simulink model "SimLink04"  (R2021a)
settings: Solver=VariableStepAuto  StartTime=0.0  StopTime=10.0  RelTol=1e-3
libraries: dsparch4 x1, simulink_extras x1
settings Model: Creator=lefs3303  LastModifiedBy=lefs3303

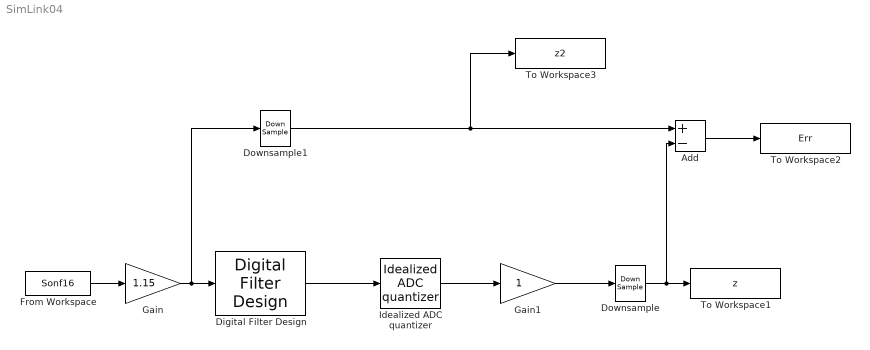
== system SimLink04 ==
  Add : Sum  Inputs=+-
  Digital Filter Design : dsparch4/Digital Filter Design  mwdsp_browser_bugfix_var=off
  Downsample : DownSample  RateOptions=Allow multirate processing
  Downsample1 : DownSample  RateOptions=Allow multirate processing
  From Workspace : FromWorkspace  VariableName=Sonf16  SampleTime=1/16000
  Gain : Gain  Gain=1.15
  Gain1 : Gain
  Idealized ADC quantizer : simulink_extras/Additional Discrete/Idealized ADC quantizer  NumberOfConverterBits=8  Vmin=-1  Vmax=1  OutputDataType=double  OutputNegativeValues=on
  To Workspace1 : ToWorkspace  VariableName=z  SampleTime=-1
      settings: Save2DSignal=2-D array (concatenate along first dimension)
  To Workspace2 : ToWorkspace  VariableName=Err  SampleTime=-1
      settings: Save2DSignal=2-D array (concatenate along first dimension)
  To Workspace3 : ToWorkspace  VariableName=z2  SampleTime=-1
      settings: Save2DSignal=2-D array (concatenate along first dimension)
  wires:
  From Workspace/1 -> Gain/1
  Gain/1 -> Downsample1/1, Digital Filter Design/1
  Digital Filter Design/1 -> Idealized ADC quantizer/1
  Idealized ADC quantizer/1 -> Gain1/1
  Gain1/1 -> Downsample/1
  Downsample/1 -> Add/2, To Workspace1/1
  Downsample1/1 -> To Workspace3/1, Add/1
  Add/1 -> To Workspace2/1
